simulink model "matrixinv"  (Simulink 6.6)
settings: Solver=FixedStepDiscrete  StartTime=0.0  StopTime=10.0  FixedStep=1  RelTol=1e-3
settings Model: Creator=ksmyth  LastModifiedBy=ksmyth

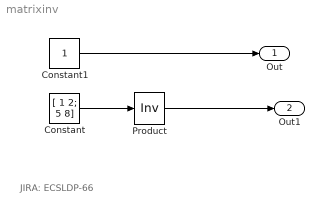
== system matrixinv ==
  note: JIRA: ECSLDP-66
  Constant : Constant  Value=[ 1 2; 5 8]
  Constant1 : Constant
  Product : Product  Inputs=/  Multiplication=Matrix(*)  RndMeth=Zero
  Out : Outport
  Out1 : Outport  Port=2
  wires:
  Constant/1 -> Product/1
  Product/1 -> Out1/1
  Constant1/1 -> Out/1
